simulink model "com_trajectory_gen"  (Simulink 10.2)
settings: Solver=FixedStepDiscrete  StartTime=0.0  StopTime=Pctrl.par.Tsim  FixedStep=Ts  RelTol=1e-3  EnableMultiTasking=on
values from neighbouring files (symbols this model uses):
  Pctrl = calculate_preview(Zdes, Tsample, Tpre, Tsim)    [sample_pattern_gen.m]
settings Model: Creator=henz_be  LastModifiedBy=isclab
settings DataIOCC: LimitDataPoints=on
settings OptimizationCC: InitFltsAndDblsToZero=on
settings DebuggingCC: SaveWithParameterizedLinksMsg=none  UnderspecifiedInitializationDetection=Simplified  SignalResolutionControl=TryResolveAllWithWarning  SolverPrmCheckMsg=warning  MultiTaskDSMMsg=warning  MultiTaskCondExecSysMsg=none
settings GRTTargetCC: TargetFcnLib=ansi_tfl_tmw.mat

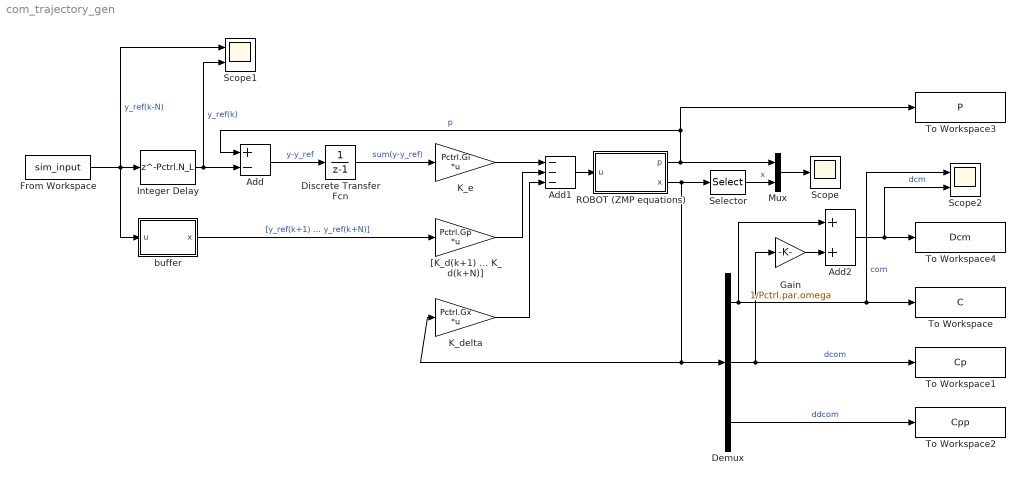
== system com_trajectory_gen ==
  Add : Sum  Inputs=+-
  Add1 : Sum  Inputs=---
  Add2 : Sum
  Demux : Demux  Outputs=3
  Discrete Transfer Fcn : DiscreteTransferFcn  Denominator=[1 -1]  SampleTime=Pctrl.Ts
  From Workspace : FromWorkspace  VariableName=sim_input  SampleTime=Pctrl.Ts  OutputAfterFinalValue=Holding final value
  Gain : Gain  Gain=1/Pctrl.par.omega
  Integer Delay : Delay  DelayLength=Pctrl.N_L  SampleTime=Pctrl.Ts
  K_delta : Gain  Gain=Pctrl.Gx  Multiplication=Matrix(K*u)
  K_e : Gain  Gain=Pctrl.Gi  Multiplication=Matrix(K*u)
  Mux : Mux  Inputs=2
  ROBOT (ZMP equations) : Subsystem
  Scope : Scope
  Scope1 : Scope  NumInputPorts=2
  Scope2 : Scope  NumInputPorts=2
  Selector : Selector  InputPortWidth=3  IndexOptions=Index vector (dialog)  Indices=1  OutputSizes=1
  To Workspace : ToWorkspace  VariableName=C  SaveFormat=Timeseries  SampleTime=Pctrl.Ts
  To Workspace1 : ToWorkspace  VariableName=Cp  SaveFormat=Timeseries  SampleTime=Pctrl.Ts
  To Workspace2 : ToWorkspace  VariableName=Cpp  SaveFormat=Timeseries  SampleTime=Pctrl.Ts
  To Workspace3 : ToWorkspace  VariableName=P  SaveFormat=Timeseries  SampleTime=Pctrl.Ts
  To Workspace4 : ToWorkspace  VariableName=Dcm  SaveFormat=Timeseries  SampleTime=Pctrl.Ts
  "[K_d(k+1) ... K_d(k+N)]" : Gain  Gain=Pctrl.Gp  Multiplication=Matrix(K*u)
  buffer : Subsystem
  wires:
  ROBOT (ZMP equations)/1(p) -> Add/1, To Workspace3/1, Mux/1  "p"
  Add1/1 -> ROBOT (ZMP equations)/1(u)
  Integer Delay/1 -> Scope1/2, Add/2  "y_ref(k)"
  ROBOT (ZMP equations)/2(x) -> K_delta/1, Demux/1, Selector/1
  Add/1 -> Discrete Transfer Fcn/1  "y-y_ref"
  Discrete Transfer Fcn/1 -> K_e/1  "sum(y-y_ref)"
  K_e/1 -> Add1/1
  buffer/1(x) -> "[K_d(k+1) ... K_d(k+N)]"/1  "[y_ref(k+1) ... y_ref(k+N)]"
  Selector/1 -> Mux/2  "x"
  Mux/1 -> Scope/1
  From Workspace/1 -> buffer/1(u), Scope1/1, Integer Delay/1  "y_ref(k-N)"
  "[K_d(k+1) ... K_d(k+N)]"/1 -> Add1/2
  K_delta/1 -> Add1/3
  Demux/1 -> Add2/1, Scope2/1, To Workspace/1  "com"
  Demux/2 -> Gain/1, To Workspace1/1  "dcom"
  Demux/3 -> To Workspace2/1  "ddcom"
  Gain/1 -> Add2/2
  Add2/1 -> Scope2/2, To Workspace4/1  "dcm"

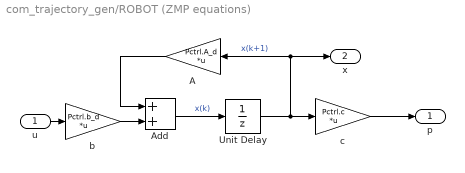
== system com_trajectory_gen/ROBOT (ZMP equations) ==
  u : Inport
  A : Gain  Gain=Pctrl.A_d  Multiplication=Matrix(K*u)
  Add : Sum
  Unit Delay : UnitDelay  InitialCondition=[0,0,0]  SampleTime=Pctrl.Ts  HasFrameUpgradeWarning=on
  b : Gain  Gain=Pctrl.b_d  Multiplication=Matrix(K*u)
  c : Gain  Gain=Pctrl.c  Multiplication=Matrix(K*u)
  p : Outport
  x : Outport  Port=2
  wires:
  b/1 -> Add/2
  Add/1 -> Unit Delay/1  "x(k)"
  A/1 -> Add/1
  Unit Delay/1 -> c/1, A/1, x/1  "x(k+1)"
  u/1 -> b/1
  c/1 -> p/1

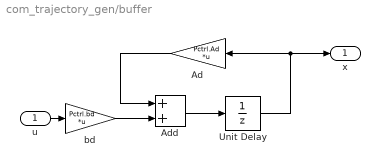
== system com_trajectory_gen/buffer ==
  u : Inport
  Ad : Gain  Gain=Pctrl.Ad  Multiplication=Matrix(K*u)
  Add : Sum
  Unit Delay : UnitDelay  SampleTime=Pctrl.Ts  HasFrameUpgradeWarning=on
  bd : Gain  Gain=Pctrl.bd  Multiplication=Matrix(K*u)
  x : Outport
  wires:
  u/1 -> bd/1
  Unit Delay/1 -> x/1, Ad/1
  Ad/1 -> Add/1
  Add/1 -> Unit Delay/1
  bd/1 -> Add/2
